simulink model "STMPPT"  (R2023a)
settings: Solver=FixedStepAuto  StartTime=0.0  StopTime=1.0  MaxStep=1e-4  RelTol=1e-3
undefined symbols (not defined in the file): Acid, Lead, sigbuilder_block, Slope_Vdc, Ts
libraries: sldrtlib x8, spsDiodeLib x7, spsPVArrayLib x7, spsSeriesRLCBranchLib x4, spspowerguiLib x2, spsBatteryLib x1, spsCurrentMeasurementLib x1, spsMosfetLib x1, spsPWMGeneratorDCDCLib x1, spsVoltageMeasurementLib x1, spsControlledVoltageSourceLib x1, simulink x1
settings Model: Creator=Asma Ul Husna  LastModifiedBy=HP
settings SolverCC: AlgebraicLoopSolver=TrustRegion
settings DataIOCC: ReturnWorkspaceOutputs=off
settings DebuggingCC: UnconnectedInputMsg=warning  UnconnectedOutputMsg=warning  UnconnectedLineMsg=warning  ArithmeticOperatorsInVariantConditions=warning
settings ModelReferenceCC: EnableRefExpFcnMdlSchedulingChecks=on
settings SFSimCC: SimUseLocalCustomCode=off  CustomCodeUndefinedFunction=UseInterfaceOnly
settings RTWCC: RTWUseLocalCustomCode=off  DLArmComputeVersion=19.05
settings CodeAppCC: StateflowObjectComments=on
settings SimscapeCC: SimscapeNormalizeSystem=off

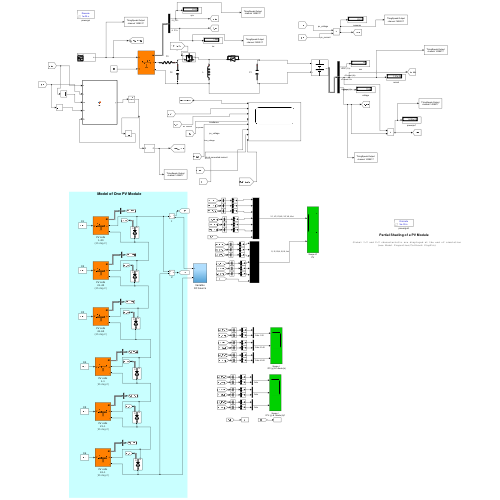
[thumbnail: Simulink's stored preview of the top-level diagram]
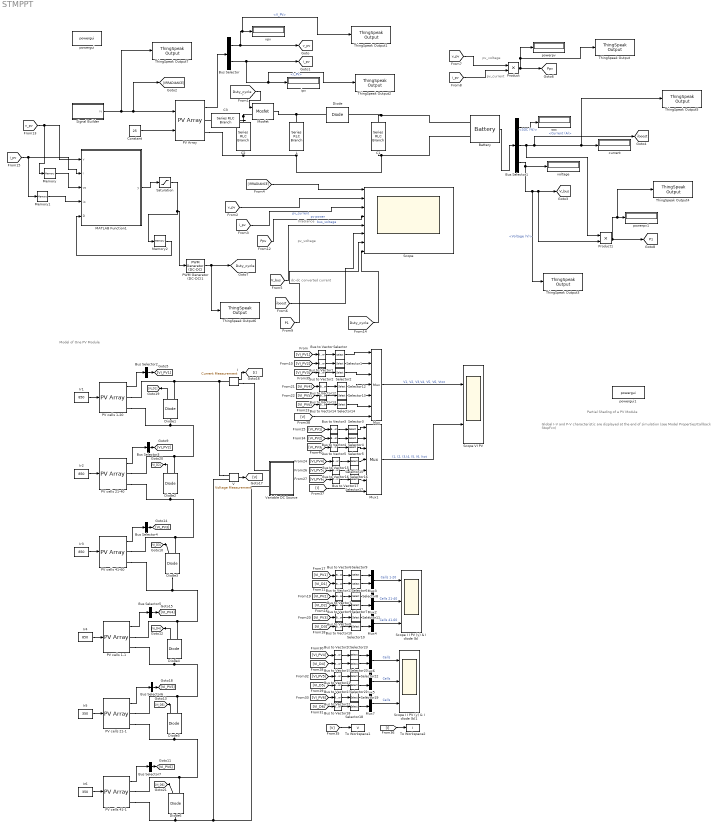
== system STMPPT ==
  note: dc-dc converted current
  note: pv_voltage
  note: r
  note: Irradiance
  note: pv_voltage
  note: pv_current
  note: Model of One PV Module
  note: Partial Shading of a PV Module
  note: Global I-V and P-V characteristic are displayed at the end of simulation
      | (see Model Properties/Callback StopFcn)
  Battery : spsBatteryLib/Battery  BatType=Lead-Acid  ShowTempParam=off  ThermalPreset=no  ShowAgeParam=off  NomV=12  NomQ=100  SOC=45  Batt_Tr=1  PresetModel=on  MaxQ=104.1667  MinV=9  FullV=13.0658  Dis_rate=20  R=0.0012  Normal_OP=31.0278  expZone="[12.2171     0.333333]"  current=[6.5 13 32.5]  Units=Time  Tci=20  NomT=20  T2=-30  MaxQ2=4.8  FullV2=7.1  Normal_OP2=5.655  expZone2="[6.58           1]"  Rca=0.6  ti=2000  Dp=0  Neq0=0  Tsim=1e6  Ta1=25  Qeol=5.4*0.9  Reol=0.013333*1.2  Char_age=[2.3478, 3]  Dis_age=[2.3478, 10]  N1=1500  N2=10500  N3=1000  N4=1400  Ta2=45  N5=950
  Bus Selector : BusSelector  OutputSignals=V_PV,I_PV
  Bus Selector1 : BusSelector  OutputSignals=SOC (%),Current (A),Voltage (V)
  Bus Selector{2..7} (6 alike) : BusSelector  OutputSignals=V_PV,I_PV  OutputAsBus=on
  Bus to Vector{,1..23} (24 alike) : BusToVector
  C1 : spsSeriesRLCBranchLib/Series RLC Branch  LConnTagsString=__new0  RConnTagsString=__new0  BranchType=C  Resistance=1  Inductance=1e-3  SetiL0=off  InitialCurrent=0  Capacitance=1.850e-6  Setx0=off  InitialVoltage=0  Measurements=None
  C2 : spsSeriesRLCBranchLib/Series RLC Branch  LConnTagsString=__new0  RConnTagsString=__new0  BranchType=C  Resistance=0.001  Inductance=1e-3  SetiL0=off  InitialCurrent=0  Capacitance=1000e-6  Setx0=off  InitialVoltage=0  Measurements=None
  C3 : spsSeriesRLCBranchLib/Series RLC Branch  LConnTagsString=__new0  RConnTagsString=__new0  BranchType=R  Resistance=0.0001  Inductance=1e-3  SetiL0=off  InitialCurrent=0  Capacitance=1000e-6  Setx0=off  InitialVoltage=0  Measurements=None
  Constant : Constant  Value=25
  Diode : spsDiodeLib/Diode  Ron=0.001  Lon=0  Vf=0.8  IC=0  UseSnubber=0  Rs=500  Cs=250e-9  Measurements=off
  Diode{1..6} (6 alike) : spsDiodeLib/Diode  Ron=0.001  Lon=0  Vf=0.7  IC=0  UseSnubber=off  Rs=1e5*inf  Cs=inf  Measurements=on
  I : spsCurrentMeasurementLib/Current Measurement  PhasorSimulation=off  OutputType=Complex  PSBequivalent=0
  Ir{1..4} (4 alike) : Constant  Value=850
  Ir5 : Constant  Value=350
  Ir6 : Constant  Value=350
  L : spsSeriesRLCBranchLib/Series RLC Branch  LConnTagsString=__new0  RConnTagsString=__new0  BranchType=L  Resistance=1  Inductance=1.92e-6  SetiL0=off  InitialCurrent=0  Capacitance=1e-6  Setx0=off  InitialVoltage=0  Measurements=None
  MATLAB Function1 : MATLAB Function  TreatAsAtomicUnit=on
  Memory : Memory
  Memory1 : Memory
  Memory2 : Memory
  Mosfet : spsMosfetLib/Mosfet  Ron=0.1  Lon=0  Rd=0.01  Vfd=0  IC=0  Rs=1e5  Cs=inf  Measurements=off
  Mux : Mux  Inputs=7
  Mux1 : Mux  Inputs=7
  Mux{2..7} (6 alike) : Mux  Inputs=2
  PV Array : spsPVArrayLib/PV Array  Npar=1  Nser=1  PlotType=one module @ 25 deg.C & specified irradiances  S_vec="[ 1000  500  100 ]"  Temp_C_vec="[ 45 25  ]"  ModuleName=User-defined  PlotWhenSelected=off  Pm=213.15  Ncell=60  Voc=36.3  Isc=7.84  Vm=29  Im=7.35  beta_Voc_pc=-0.36099  alpha_Isc_pc=0.102  beta_Voc=-0.13104  alpha_Isc=0.0079968  IL=7.8654  I0=2.9273e-10  nI=0.98119  Rsh=313.0553  Rs=0.39381  RobustModel=off  RobustCellTemperature=313.3991  BAL=on  Tc=1e-6  Tfilter=5e-5
  PV cells 1-1 : spsPVArrayLib/PV Array  Npar=1  Nser=1  PlotType=array @ 25 deg.C & specified irradiances  S_vec="[ 1000  300  600 ]"  Temp_C_vec="[ 45 25  ]"  ModuleName=User-defined  PlotWhenSelected=off  Pm=83.2824  Ncell=60/3  Voc=37.92*20/60  Isc=8.62  Vm=30.96*20/60  Im=8.07  beta_Voc_pc=-0.33969  alpha_Isc_pc=0.063701  beta_Voc=-0.042937  alpha_Isc=0.005491  IL=8.6307  I0=1.4176e-10  nI=0.99132  Rsh=82.1161  Rs=0.098625  RobustModel=on  RobustCellTemperature=25  BAL=on  Tc=1e-5  Tfilter=5e-5
      settings: AttributesFormatString=(%<RobustCellTemperature> deg.C)
  PV cells 1-20 : spsPVArrayLib/PV Array  Npar=1  Nser=1  PlotType=array @ 25 deg.C & specified irradiances  S_vec="[ 1000  300  600 ]"  Temp_C_vec="[ 45 25  ]"  ModuleName=User-defined  PlotWhenSelected=off  Pm=83.2824  Ncell=60/3  Voc=37.92*20/60  Isc=8.62  Vm=30.96*20/60  Im=8.07  beta_Voc_pc=-0.33969  alpha_Isc_pc=0.063701  beta_Voc=-0.042937  alpha_Isc=0.005491  IL=8.6307  I0=1.4176e-10  nI=0.99132  Rsh=82.1161  Rs=0.098625  RobustModel=on  RobustCellTemperature=25  BAL=on  Tc=1e-5  Tfilter=5e-5
      settings: AttributesFormatString=(%<RobustCellTemperature> deg.C)
  PV cells 21-1 : spsPVArrayLib/PV Array  Npar=1  Nser=1  PlotType=array @ 25 deg.C & specified irradiances  S_vec="[ 1000  300  600 ]"  Temp_C_vec="[ 45 25  ]"  ModuleName=User-defined  PlotWhenSelected=off  Pm=83.2824  Ncell=60/3  Voc=37.92*20/60  Isc=8.62  Vm=30.96*20/60  Im=8.07  beta_Voc_pc=-0.33969  alpha_Isc_pc=0.063701  beta_Voc=-0.042937  alpha_Isc=0.005491  IL=8.6307  I0=1.4176e-10  nI=0.99132  Rsh=82.1161  Rs=0.098625  RobustModel=on  RobustCellTemperature=25  BAL=on  Tc=1e-5  Tfilter=5e-5
      settings: AttributesFormatString=(%<RobustCellTemperature> deg.C)
  PV cells 21-40 : spsPVArrayLib/PV Array  Npar=1  Nser=1  PlotType=array @ 25 deg.C & specified irradiances  S_vec="[ 1000  300  600 ]"  Temp_C_vec="[ 45 25  ]"  ModuleName=User-defined  PlotWhenSelected=off  Pm=83.2824  Ncell=60/3  Voc=37.92*20/60  Isc=8.62  Vm=30.96*20/60  Im=8.07  beta_Voc_pc=-0.33969  alpha_Isc_pc=0.063701  beta_Voc=-0.042937  alpha_Isc=0.005491  IL=8.6307  I0=1.4176e-10  nI=0.99132  Rsh=82.1161  Rs=0.098625  RobustModel=on  RobustCellTemperature=25  BAL=on  Tc=1e-5  Tfilter=5e-5
      settings: AttributesFormatString=(%<RobustCellTemperature> deg.C)
  PV cells 41-1 : spsPVArrayLib/PV Array  Npar=1  Nser=1  PlotType=array @ 25 deg.C & specified irradiances  S_vec="[ 1000  300  600 ]"  Temp_C_vec="[ 45 25  ]"  ModuleName=User-defined  PlotWhenSelected=off  Pm=83.2824  Ncell=60/3  Voc=37.92*20/60  Isc=8.62  Vm=30.96*20/60  Im=8.07  beta_Voc_pc=-0.33969  alpha_Isc_pc=0.063701  beta_Voc=-0.042937  alpha_Isc=0.005491  IL=8.6307  I0=1.4176e-10  nI=0.99132  Rsh=82.1161  Rs=0.098625  RobustModel=on  RobustCellTemperature=25  BAL=on  Tc=1e-5  Tfilter=5e-5
      settings: AttributesFormatString=(%<RobustCellTemperature> deg.C)
  PV cells 41-60 : spsPVArrayLib/PV Array  Npar=1  Nser=1  PlotType=array @ 25 deg.C & specified irradiances  S_vec="[ 1000  300  600 ]"  Temp_C_vec="[ 45 25  ]"  ModuleName=User-defined  PlotWhenSelected=off  Pm=83.2824  Ncell=60/3  Voc=37.92*20/60  Isc=8.62  Vm=30.96*20/60  Im=8.07  beta_Voc_pc=-0.33969  alpha_Isc_pc=0.063701  beta_Voc=-0.042937  alpha_Isc=0.005491  IL=8.6307  I0=1.4176e-10  nI=0.99132  Rsh=82.1161  Rs=0.098625  RobustModel=on  RobustCellTemperature=25  BAL=on  Tc=1e-5  Tfilter=5e-5
      settings: AttributesFormatString=(%<RobustCellTemperature> deg.C)
  PWM Generator (DC-DC)1 : spsPWMGeneratorDCDCLib/PWM Generator (DC-DC)  Fsw=30000  Ts=10e-6
  Product : Product
  Product1 : Product
  Saturation : Saturate  UpperLimit=0.9  LowerLimit=0
  Scope : Scope  NumInputPorts=8
  Scope I I PV (y) & I diode (b) : Scope  NumInputPorts=3
  Scope I I PV (y) & I diode (b)1 : Scope  NumInputPorts=3
  Scope VI PV : Scope  NumInputPorts=2
  Selector{,1..2,6..7,10,12..14,18,20..21} (12 alike) : Selector  InputPortWidth=2  IndexOptions=Index vector (dialog)  Indices=[1]  OutputSizes=1
  Selector{3..5,8..9,11,15..17,19,22..23} (12 alike) : Selector  InputPortWidth=2  IndexOptions=Index vector (dialog)  Indices=[2]  OutputSizes=1
  Signal Builder : Subsystem  Tag=STV Subsys  LoadFcn=sigbuilder_block('load');  StartFcn=sigbuilder_block('start');  StopFcn=sigbuilder_block('stop');  ClipboardFcn=sigbuilder_block('clipboard');  mask(Sigbuilder block){tuvar=[0:10]}
      mask help: Simulink:masks:SigbuilderBlock_MD
      mask init:
      | if ~strcmp(get_param(bdroot(gcbh),'SimulationStatus'),'stopped') tuvar = sigbuilder_block('maskInit'); end
      settings: CopyFcn=sigbuilder_block('copy');  DeleteFcn=sigbuilder_block('delete');  ModelCloseFcn=sigbuilder_block('modelClose');  PreSaveFcn=sigbuilder_block('preSave');  PauseFcn=sigbuilder_block('pause');  ContinueFcn=sigbuilder_block('continue');  NameChangeFcn=sigbuilder_block('namechange');  OpenFcn=sigbuilder_block('open',[437.6 199.2 550.4 400 ]);  CloseFcn=sigbuilder_block('close');
      mask Display: plot(0, 0, 100, 100,[2, 2, 32, 32, 2], [68, 8, 8, 68, 68],[32, 2], [38, 38], [32, 19, 2],[53, 60, 44], [32, 17, 17, 2],[16, 16, 31, 31]);txt = getActiveGroup(gcbh);text(2, 100, txt,'verticalAlignment', 'top');
  ThingSpeak Output : sldrtlib/Internet of Things/ThingSpeak Output  DrvAddress=1428517  DrvOptions=[1 20 67 82 53 74 88 49 56 84 88 56 85 69 66 75 87 87 97 112 105 46 116 104 105 110 103 115 112 101 97 107 46 99 111 109 0 0 0 0 0 0 0 0 0 0 0 0 0 0 0 0 0 0 0 0 0 0 0 0 0 0 0 0 0 0 0 0 0 0 0 0 0 0 0 0 0 0 0 0 0 0 0 0 0 0 0 0 0 0 0 0 0 0 0 0 0 0 0 0 0 0 0 0 0 0 0 0 0 0 0 0 0 0 0 0 0 0 0 0 0 0 0 0 0 0 0 0 0 0 0 0 0 0 0 0 0 0 0 0 0 0 0 0 0 0 0 0 0 0 0 0 0 0 0 0 0 0 0 0 0 0 0 0 0 0 0 0 0 0 0 0 0 0 0 0 0 0 0 0 0 0 0 0 0 0 0 0 0 0 0 0 0 0 0 0 0 0 0 0 0 0 0 0 0 0 0 0 0 0 0 0 0 0 0 0 0 0 0 0 0 0 0 0 0 0 0 0 0 0 0 0 0 0 0 0 0 0 0 0 0 0 0 0 0 0 0 0 0 0 0 0 0 0 0 0]  SampleTime=0.1  MaxMissedTicks=20  ShowMissedTicks=off  YieldWhenWaiting=off  ChannelFields=4  OptParam=0  InitialValue=[]  FinalValue=[]
  ThingSpeak Output1 : sldrtlib/Internet of Things/ThingSpeak Output  DrvAddress=1428517  DrvOptions=[1 20 67 82 53 74 88 49 56 84 88 56 85 69 66 75 87 87 97 112 105 46 116 104 105 110 103 115 112 101 97 107 46 99 111 109 0 0 0 0 0 0 0 0 0 0 0 0 0 0 0 0 0 0 0 0 0 0 0 0 0 0 0 0 0 0 0 0 0 0 0 0 0 0 0 0 0 0 0 0 0 0 0 0 0 0 0 0 0 0 0 0 0 0 0 0 0 0 0 0 0 0 0 0 0 0 0 0 0 0 0 0 0 0 0 0 0 0 0 0 0 0 0 0 0 0 0 0 0 0 0 0 0 0 0 0 0 0 0 0 0 0 0 0 0 0 0 0 0 0 0 0 0 0 0 0 0 0 0 0 0 0 0 0 0 0 0 0 0 0 0 0 0 0 0 0 0 0 0 0 0 0 0 0 0 0 0 0 0 0 0 0 0 0 0 0 0 0 0 0 0 0 0 0 0 0 0 0 0 0 0 0 0 0 0 0 0 0 0 0 0 0 0 0 0 0 0 0 0 0 0 0 0 0 0 0 0 0 0 0 0 0 0 0 0 0 0 0 0 0 0 0 0 0 0 0]  SampleTime=0.1  MaxMissedTicks=20  ShowMissedTicks=off  YieldWhenWaiting=off  ChannelFields=2  OptParam=0  InitialValue=[]  FinalValue=[]
  ThingSpeak Output2 : sldrtlib/Internet of Things/ThingSpeak Output  DrvAddress=1428517  DrvOptions=[1 20 67 82 53 74 88 49 56 84 88 56 85 69 66 75 87 87 97 112 105 46 116 104 105 110 103 115 112 101 97 107 46 99 111 109 0 0 0 0 0 0 0 0 0 0 0 0 0 0 0 0 0 0 0 0 0 0 0 0 0 0 0 0 0 0 0 0 0 0 0 0 0 0 0 0 0 0 0 0 0 0 0 0 0 0 0 0 0 0 0 0 0 0 0 0 0 0 0 0 0 0 0 0 0 0 0 0 0 0 0 0 0 0 0 0 0 0 0 0 0 0 0 0 0 0 0 0 0 0 0 0 0 0 0 0 0 0 0 0 0 0 0 0 0 0 0 0 0 0 0 0 0 0 0 0 0 0 0 0 0 0 0 0 0 0 0 0 0 0 0 0 0 0 0 0 0 0 0 0 0 0 0 0 0 0 0 0 0 0 0 0 0 0 0 0 0 0 0 0 0 0 0 0 0 0 0 0 0 0 0 0 0 0 0 0 0 0 0 0 0 0 0 0 0 0 0 0 0 0 0 0 0 0 0 0 0 0 0 0 0 0 0 0 0 0 0 0 0 0 0 0 0 0 0 0]  SampleTime=0.1  MaxMissedTicks=20  ShowMissedTicks=off  YieldWhenWaiting=off  ChannelFields=3  OptParam=0  InitialValue=[]  FinalValue=[]
  ThingSpeak Output3 : sldrtlib/Internet of Things/ThingSpeak Output  DrvAddress=1428517  DrvOptions=[1 20 67 82 53 74 88 49 56 84 88 56 85 69 66 75 87 87 97 112 105 46 116 104 105 110 103 115 112 101 97 107 46 99 111 109 0 0 0 0 0 0 0 0 0 0 0 0 0 0 0 0 0 0 0 0 0 0 0 0 0 0 0 0 0 0 0 0 0 0 0 0 0 0 0 0 0 0 0 0 0 0 0 0 0 0 0 0 0 0 0 0 0 0 0 0 0 0 0 0 0 0 0 0 0 0 0 0 0 0 0 0 0 0 0 0 0 0 0 0 0 0 0 0 0 0 0 0 0 0 0 0 0 0 0 0 0 0 0 0 0 0 0 0 0 0 0 0 0 0 0 0 0 0 0 0 0 0 0 0 0 0 0 0 0 0 0 0 0 0 0 0 0 0 0 0 0 0 0 0 0 0 0 0 0 0 0 0 0 0 0 0 0 0 0 0 0 0 0 0 0 0 0 0 0 0 0 0 0 0 0 0 0 0 0 0 0 0 0 0 0 0 0 0 0 0 0 0 0 0 0 0 0 0 0 0 0 0 0 0 0 0 0 0 0 0 0 0 0 0 0 0 0 0 0 0]  SampleTime=0.1  MaxMissedTicks=20  ShowMissedTicks=off  YieldWhenWaiting=off  ChannelFields=5  OptParam=0  InitialValue=[]  FinalValue=[]
  ThingSpeak Output4 : sldrtlib/Internet of Things/ThingSpeak Output  DrvAddress=1428517  DrvOptions=[1 20 67 82 53 74 88 49 56 84 88 56 85 69 66 75 87 87 97 112 105 46 116 104 105 110 103 115 112 101 97 107 46 99 111 109 0 0 0 0 0 0 0 0 0 0 0 0 0 0 0 0 0 0 0 0 0 0 0 0 0 0 0 0 0 0 0 0 0 0 0 0 0 0 0 0 0 0 0 0 0 0 0 0 0 0 0 0 0 0 0 0 0 0 0 0 0 0 0 0 0 0 0 0 0 0 0 0 0 0 0 0 0 0 0 0 0 0 0 0 0 0 0 0 0 0 0 0 0 0 0 0 0 0 0 0 0 0 0 0 0 0 0 0 0 0 0 0 0 0 0 0 0 0 0 0 0 0 0 0 0 0 0 0 0 0 0 0 0 0 0 0 0 0 0 0 0 0 0 0 0 0 0 0 0 0 0 0 0 0 0 0 0 0 0 0 0 0 0 0 0 0 0 0 0 0 0 0 0 0 0 0 0 0 0 0 0 0 0 0 0 0 0 0 0 0 0 0 0 0 0 0 0 0 0 0 0 0 0 0 0 0 0 0 0 0 0 0 0 0 0 0 0 0 0 0]  SampleTime=0.1  MaxMissedTicks=20  ShowMissedTicks=off  YieldWhenWaiting=off  ChannelFields=7  OptParam=0  InitialValue=[]  FinalValue=[]
  ThingSpeak Output5 : sldrtlib/Internet of Things/ThingSpeak Output  DrvAddress=1428517  DrvOptions=[1 20 67 82 53 74 88 49 56 84 88 56 85 69 66 75 87 87 97 112 105 46 116 104 105 110 103 115 112 101 97 107 46 99 111 109 0 0 0 0 0 0 0 0 0 0 0 0 0 0 0 0 0 0 0 0 0 0 0 0 0 0 0 0 0 0 0 0 0 0 0 0 0 0 0 0 0 0 0 0 0 0 0 0 0 0 0 0 0 0 0 0 0 0 0 0 0 0 0 0 0 0 0 0 0 0 0 0 0 0 0 0 0 0 0 0 0 0 0 0 0 0 0 0 0 0 0 0 0 0 0 0 0 0 0 0 0 0 0 0 0 0 0 0 0 0 0 0 0 0 0 0 0 0 0 0 0 0 0 0 0 0 0 0 0 0 0 0 0 0 0 0 0 0 0 0 0 0 0 0 0 0 0 0 0 0 0 0 0 0 0 0 0 0 0 0 0 0 0 0 0 0 0 0 0 0 0 0 0 0 0 0 0 0 0 0 0 0 0 0 0 0 0 0 0 0 0 0 0 0 0 0 0 0 0 0 0 0 0 0 0 0 0 0 0 0 0 0 0 0 0 0 0 0 0 0]  SampleTime=0.1  MaxMissedTicks=20  ShowMissedTicks=off  YieldWhenWaiting=off  ChannelFields=6  OptParam=0  InitialValue=[]  FinalValue=[]
  ThingSpeak Output6 : sldrtlib/Internet of Things/ThingSpeak Output  DrvAddress=1428517  DrvOptions=[1 20 67 82 53 74 88 49 56 84 88 56 85 69 66 75 87 87 97 112 105 46 116 104 105 110 103 115 112 101 97 107 46 99 111 109 0 0 0 0 0 0 0 0 0 0 0 0 0 0 0 0 0 0 0 0 0 0 0 0 0 0 0 0 0 0 0 0 0 0 0 0 0 0 0 0 0 0 0 0 0 0 0 0 0 0 0 0 0 0 0 0 0 0 0 0 0 0 0 0 0 0 0 0 0 0 0 0 0 0 0 0 0 0 0 0 0 0 0 0 0 0 0 0 0 0 0 0 0 0 0 0 0 0 0 0 0 0 0 0 0 0 0 0 0 0 0 0 0 0 0 0 0 0 0 0 0 0 0 0 0 0 0 0 0 0 0 0 0 0 0 0 0 0 0 0 0 0 0 0 0 0 0 0 0 0 0 0 0 0 0 0 0 0 0 0 0 0 0 0 0 0 0 0 0 0 0 0 0 0 0 0 0 0 0 0 0 0 0 0 0 0 0 0 0 0 0 0 0 0 0 0 0 0 0 0 0 0 0 0 0 0 0 0 0 0 0 0 0 0 0 0 0 0 0 0]  SampleTime=0.1  MaxMissedTicks=20  ShowMissedTicks=off  YieldWhenWaiting=off  ChannelFields=8  OptParam=0  InitialValue=[]  FinalValue=[]
  ThingSpeak Output7 : sldrtlib/Internet of Things/ThingSpeak Output  DrvAddress=1428517  DrvOptions=[1 20 67 82 53 74 88 49 56 84 88 56 85 69 66 75 87 87 97 112 105 46 116 104 105 110 103 115 112 101 97 107 46 99 111 109 0 0 0 0 0 0 0 0 0 0 0 0 0 0 0 0 0 0 0 0 0 0 0 0 0 0 0 0 0 0 0 0 0 0 0 0 0 0 0 0 0 0 0 0 0 0 0 0 0 0 0 0 0 0 0 0 0 0 0 0 0 0 0 0 0 0 0 0 0 0 0 0 0 0 0 0 0 0 0 0 0 0 0 0 0 0 0 0 0 0 0 0 0 0 0 0 0 0 0 0 0 0 0 0 0 0 0 0 0 0 0 0 0 0 0 0 0 0 0 0 0 0 0 0 0 0 0 0 0 0 0 0 0 0 0 0 0 0 0 0 0 0 0 0 0 0 0 0 0 0 0 0 0 0 0 0 0 0 0 0 0 0 0 0 0 0 0 0 0 0 0 0 0 0 0 0 0 0 0 0 0 0 0 0 0 0 0 0 0 0 0 0 0 0 0 0 0 0 0 0 0 0 0 0 0 0 0 0 0 0 0 0 0 0 0 0 0 0 0 0]  SampleTime=0.1  MaxMissedTicks=20  ShowMissedTicks=off  YieldWhenWaiting=off  ChannelFields=1  OptParam=0  InitialValue=[]  FinalValue=[]
  To Workspace1 : ToWorkspace  VariableName=V  SampleTime=1e-3
  To Workspace2 : ToWorkspace  VariableName=I  SampleTime=1e-3
  V : spsVoltageMeasurementLib/Voltage Measurement  PhasorSimulation=off  OutputType=Complex  PSBequivalent=0
  Variable DC Source : Subsystem
  current : Display
  ipv : Display
  powergui : spspowerguiLib/powergui  Priority=1  SimulationMode=Discrete  SampleTime=10e-6  frequency=60  Iterations=50  frequencyindice=0  Pbase=100e6  ErrMax=1e-4  UnitsV=kV  UnitsW=MW  buscounter=0  FunctionMessages=off  echomessages=off  EnableUseOfTLC=off  CurrentSourceSwitches=off  DisableSnubberDevices=off  DisableRonSwitches=off  DisableVfSwitches=off  DisplayEquations=off  AutomaticDiscreteSolvers=off  SolverType=Tustin/Backward Euler (TBE)  Interpol=off  ExternalGateDelay=off  methode=off  Ts=100  x0status=blocks  SPID=on  SwTol=0  HookPort=off  NonlinearTolerance=1e-4  nMaxIteration=100  ContinueOnMaxIteration=off  RestoreLinks=warning  ResistiveCurrentMeasurement=off  Frange=[0:2:500]  Ylog=off  Xlog=on  ShowGrid=off  save=off  variable=ZData  structure=0  ZoomFFT=off  StartTime=0.0  cycles=1  DisplayStyle=1  fundamental=60  FreqAxis=off  MaxFrequency=1000  frequencyindicesteady=1  RmsSteady=1  display=off
  powergui1 : spspowerguiLib/powergui  Priority=1  SimulationMode=Discrete  SampleTime=Ts  frequency=60  Iterations=50  frequencyindice=0  Pbase=100e6  ErrMax=1e-4  UnitsV=kV  UnitsW=MW  buscounter=0  FunctionMessages=off  echomessages=off  EnableUseOfTLC=off  CurrentSourceSwitches=on  DisableSnubberDevices=on  DisableRonSwitches=off  DisableVfSwitches=off  DisplayEquations=off  AutomaticDiscreteSolvers=off  SolverType=Tustin/Backward Euler (TBE)  Interpol=off  ExternalGateDelay=off  methode=off  Ts=0  x0status=blocks  SPID=off  SwTol=0  HookPort=off  NonlinearTolerance=1e-4  nMaxIteration=100  ContinueOnMaxIteration=off  RestoreLinks=warning  ResistiveCurrentMeasurement=off  Frange=[0:2:500]  Ylog=off  Xlog=on  ShowGrid=off  save=off  variable=ZData  structure=0  ZoomFFT=on  StartTime=0.0  cycles=1  DisplayStyle=1  fundamental=60  FreqAxis=off  MaxFrequency=1000  frequencyindicesteady=1  RmsSteady=1  display=off
  powerpv : Display
  powerpv1 : Display
  soc : Display
  "voltage " : Display
  vpv : Display
  tag scope: Duty_cycle=global, P1=global, Ppv=global, V_bus=global, i_pv=global, iboost=global, v_pv=global
  wires:
  Battery/1 -> Bus Selector1/1
  Bus Selector/2 -> ThingSpeak Output2/1, ipv/1, [i_pv]  "<I_PV>"
  Product/1 -> ThingSpeak Output/1, powerpv/1, [Ppv]
  [Duty_cycle] -> Scope/8
  Constant/1 -> PV Array/2
  Bus Selector1/2 -> Product1/1, [iboost], ThingSpeak Output5/1, current/1  "<Current (A)>"
  [v_pv] -> Product/1
  [Ppv] -> Scope/4  "pv power"
  Product1/1 -> ThingSpeak Output4/1, powerpv1/1, [P1]
  PWM Generator (DC-DC)1/1 -> ThingSpeak Output6/1, [Duty_cycle]
  Bus Selector1/1 -> soc/1  "<SOC (%)>"
  [i_pv] -> Product/2
  Bus Selector/1 -> ThingSpeak Output1/1, vpv/1, [v_pv]  "<V_PV>"
  Bus Selector1/3 -> ThingSpeak Output3/1, Product1/2, [V_bus], "voltage "/1  "<Voltage (V)>"
  [Duty_cycle] -> Mosfet/1
  [v_pv] -> Scope/2
  [IRRADIANCE] -> Scope/1
  [V_bus] -> Scope/5  "bus_voltage"
  [i_pv] -> Scope/3  "pv_current"
  PV Array/1 -> Bus Selector/1
  [iboost] -> Scope/6
  [P1] -> Scope/7
  Signal Builder/1(iv) -> ThingSpeak Output7/1, [IRRADIANCE], PV Array/1
  [v_pv] -> Memory/1, MATLAB Function1/1(v)
  Memory/1 -> MATLAB Function1/3(vo)
  [i_pv] -> Memory1/1, MATLAB Function1/2(i)
  Memory1/1 -> MATLAB Function1/4(io)
  MATLAB Function1/1(y) -> Saturation/1
  Saturation/1 -> PWM Generator (DC-DC)1/1, Memory2/1
  Memory2/1 -> MATLAB Function1/5(D)
  [VI_PV4] -> Bus to Vector12/1
  Bus to Vector13/1 -> Selector13/1
  [VI_PV5] -> Bus to Vector13/1
  Selector21/1 -> Mux5/2
  [VI_D4] -> Bus to Vector19/1
  Selector18/1 -> Mux7/2
  Bus to Vector22/1 -> Selector19/1
  [VI_PV6] -> Bus to Vector22/1
  Mux7/1 -> Scope I I PV (y) & I diode (b)1/3  "Cells"
  Bus to Vector23/1 -> Selector21/1
  Mux5/1 -> Scope I I PV (y) & I diode (b)1/2  "Cells"
  Selector23/1 -> Mux6/1
  Bus to Vector19/1 -> Selector20/1
  Selector19/1 -> Mux7/1
  Bus to Vector18/1 -> Selector18/1
  Bus to Vector20/1 -> Selector23/1
  Selector22/1 -> Mux5/1
  [V] -> Mux/7
  Selector17/1 -> Mux1/6
  Selector15/1 -> Mux1/4
  Selector16/1 -> Mux1/5
  Selector12/1 -> Mux/4
  Selector14/1 -> Mux/6
  Selector13/1 -> Mux/5
  Bus to Vector16/1 -> Selector16/1
  [VI_PV4] -> Bus to Vector15/1
  [VI_PV5] -> Bus to Vector16/1
  Bus to Vector15/1 -> Selector15/1
  [VI_D6] -> Bus to Vector18/1
  [VI_D5] -> Bus to Vector23/1
  Bus to Vector17/1 -> Selector17/1
  [I] -> Mux1/7
  Bus Selector5/1 -> [VI_PV4]
  Diode5/1 -> [VI_D5]
  Bus Selector6/1 -> [VI_PV5]
  Ir5/1 -> PV cells 21-1/1
  Ir6/1 -> PV cells 41-1/1
  [VI_PV6] -> Bus to Vector14/1
  Bus Selector7/1 -> [VI_PV6]
  PV cells 21-1/1 -> Bus Selector6/1
  Diode4/1 -> [VI_D4]
  PV cells 1-1/1 -> Bus Selector5/1
  Ir4/1 -> PV cells 1-1/1
  PV cells 41-1/1 -> Bus Selector7/1
  Diode6/1 -> [VI_D6]
  Bus to Vector11/1 -> Selector6/1
  [VI_PV2] -> Bus to Vector1/1
  Bus to Vector7/1 -> Selector8/1
  Diode1/1 -> [VI_D1]
  Selector8/1 -> Mux2/1
  Diode3/1 -> [VI_D3]
  Ir1/1 -> PV cells 1-20/1
  Selector11/1 -> Mux4/1
  Bus to Vector4/1 -> Selector4/1
  Ir2/1 -> PV cells 21-40/1
  Bus to Vector12/1 -> Selector12/1
  [VI_PV1] -> Bus to Vector6/1
  [I] -> To Workspace2/1
  Selector2/1 -> Mux/3
  Bus to Vector3/1 -> Selector3/1
  [VI_PV3] -> Bus to Vector5/1
  Mux4/1 -> Scope I I PV (y) & I diode (b)/3  "Cells 41-60"
  Bus to Vector9/1 -> Selector7/1
  Mux2/1 -> Scope I I PV (y) & I diode (b)/2  "Cells 21-40"
  Selector20/1 -> Mux6/2
  Selector6/1 -> Mux3/2
  [V] -> To Workspace1/1
  Selector/1 -> Mux/1
  Selector7/1 -> Mux2/2
  Bus to Vector21/1 -> Selector22/1
  [VI_PV5] -> Bus to Vector21/1
  Mux1/1 -> Scope VI PV/2  "I1, I2, I3,I4, I5, I6, Itot"
  [VI_PV2] -> Bus to Vector4/1
  [VI_D2] -> Bus to Vector9/1
  PV cells 41-60/1 -> Bus Selector4/1
  [VI_PV6] -> Bus to Vector17/1
  V/1 -> [V]
  Selector10/1 -> Mux4/2
  Selector9/1 -> Mux3/1
  Mux6/1 -> Scope I I PV (y) & I diode (b)1/1  "Cells"
  [VI_PV1] -> Bus to Vector3/1
  Ir3/1 -> PV cells 41-60/1
  [VI_PV3] -> Bus to Vector8/1
  Bus to Vector1/1 -> Selector1/1
  Bus to Vector6/1 -> Selector9/1
  I/1 -> [I]
  PV cells 1-20/1 -> Bus Selector2/1
  Selector1/1 -> Mux/2
  Bus to Vector/1 -> Selector/1
  Mux/1 -> Scope VI PV/1  "V1, V2, V3,V4, V5, V6, Vtot"
  [VI_PV2] -> Bus to Vector7/1
  Bus Selector3/1 -> [VI_PV2]
  Mux3/1 -> Scope I I PV (y) & I diode (b)/1  "Cells 1-20"
  [VI_PV3] -> Bus to Vector2/1
  Bus to Vector5/1 -> Selector5/1
  [VI_PV4] -> Bus to Vector20/1
  PV cells 21-40/1 -> Bus Selector3/1
  Selector3/1 -> Mux1/1
  [VI_PV1] -> Bus to Vector/1
  Bus to Vector2/1 -> Selector2/1
  Diode2/1 -> [VI_D2]
  Selector4/1 -> Mux1/2
  Bus to Vector8/1 -> Selector11/1
  Bus Selector4/1 -> [VI_PV3]
  Bus to Vector10/1 -> Selector10/1
  Selector5/1 -> Mux1/3
  Bus to Vector14/1 -> Selector14/1
  Bus Selector2/1 -> [VI_PV1]
  [VI_D1] -> Bus to Vector11/1
  [VI_D3] -> Bus to Vector10/1
  connections:
  Diode/RConn1 -- L/LConn1 -- Mosfet/RConn1
  Diode/LConn1 -- C1/LConn1 -- Battery/LConn2
  C2/LConn1 -- Mosfet/LConn1 -- C3/LConn1
  C3/RConn1 -- PV Array/RConn1
  V/LConn2 -- PV cells 41-1/RConn2 -- Diode6/LConn1 -- Variable DC Source/LConn2
  PV cells 1-1/RConn1 -- Diode3/LConn1 -- PV cells 41-60/RConn2 -- Diode4/RConn1
  Diode4/LConn1 -- PV cells 1-1/RConn2 -- PV cells 21-1/RConn1 -- Diode5/RConn1
  PV cells 21-1/RConn2 -- Diode5/LConn1 -- PV cells 41-1/RConn1 -- Diode6/RConn1
  Diode1/LConn1 -- PV cells 21-40/RConn1 -- Diode2/RConn1 -- PV cells 1-20/RConn2
  C1/RConn1 -- Battery/LConn1 -- PV Array/RConn2 -- C2/RConn1 -- L/RConn1
  PV cells 21-40/RConn2 -- Diode2/LConn1 -- PV cells 41-60/RConn1 -- Diode3/RConn1
  I/RConn1 -- Variable DC Source/LConn1
  V/LConn1 -- PV cells 1-20/RConn1 -- Diode1/RConn1 -- I/LConn1

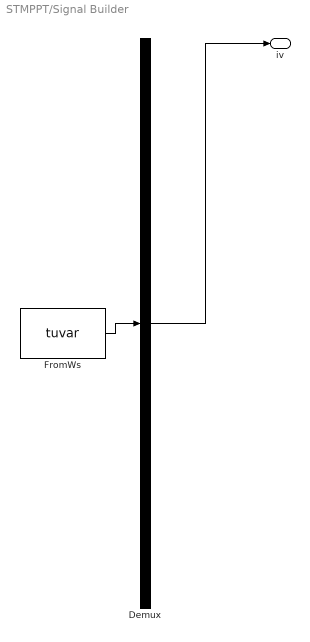
== system STMPPT/Signal Builder ==
  Demux : Demux  Tag=STV Demux  Outputs=1
      settings: DisplayOption=none
  FromWs : FromWorkspace  Tag=STV FromWs  VariableName=tuvar
      SigBuilderData=|
      | common.afterFinalStr = 'Extrapolate'
      | common.sampleTime = 0
      | dataSet.timeRange = [0 1]
      | dataSet.name = 'Sheet1'
      | sbobj.Groups.Name = 'Sheet1'
      | sbobj.Groups.Signals.Name = 'iv'
      | sbobj.Groups.Signals.XData = [0 0.1 0.2 0.2 0.3 0.4 0.5 0.6 0.7 0.8 0.8 0.9 0.9 1]
      | sbobj.Groups.Signals.YData = [25 200 390 415 655 1005 1005 725 560 475 465 405 400 140]
      | sbobj.Groups.TimeRange = [0 1]
  iv : Outport  Tag=STV Outport
  wires:
  Demux/1 -> iv/1
  FromWs/1 -> Demux/1

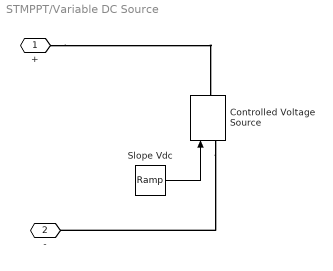
== system STMPPT/Variable DC Source ==
  Controlled Voltage Source : spsControlledVoltageSourceLib/Controlled Voltage Source  Initialize=on  Source_Type=AC  Amplitude=0  Phase=0  Frequency=0  Measurements=None
  Slope Vdc : simulink/Sources/Ramp  slope=Slope_Vdc  start=0  InitialOutput=0
  + : PMIOPort  Side=Left
  - : PMIOPort  Port=2  Side=Left
  wires:
  Slope Vdc/1 -> Controlled Voltage Source/1
  connections:
  Controlled Voltage Source/LConn1 -- -/RConn1
  +/RConn1 -- Controlled Voltage Source/RConn1

== matlab function STMPPT/MATLAB Function1 ==
  data: v input; y output; i input; vo input; io input; D input
function y = inc(v,i,vo,io,D)
m=0.6;
dv=v-vo;
di=i-io;
d=0.00004;
if dv==0
    if di==0
        m=D;
    else
        if di>0
            m=D-d;
        else
             m=D+d;
        end
    end
else
     if di/dv==-(i/v)
        m=D;
    else
        if di/dv> -(i/v)
            m=D-d;
        else
             m=D+d;
        end
     end
end
y=m;
end
